simulink model "self_triggered_mpc_simulation"  (R2023a)
settings: Solver=VariableStepAuto  StartTime=0.0  StopTime=1  RelTol=1e-3
values from neighbouring files (symbols this model uses):
  param = param_setup()    [cost_cal.m]    (also in main.m; param.mat = ; self_triggered_mpc_heemels.m)
(part 1 of 2)
settings Model: Creator=김준수  LastModifiedBy=김준수
settings DebuggingCC: UnderSpecifiedDimensionMsg=error

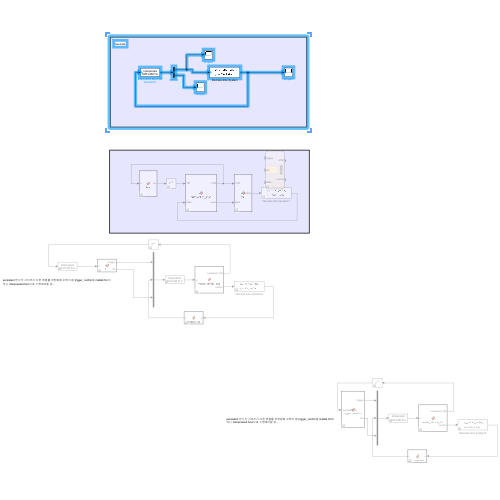
[thumbnail: Simulink's stored preview of the top-level diagram]
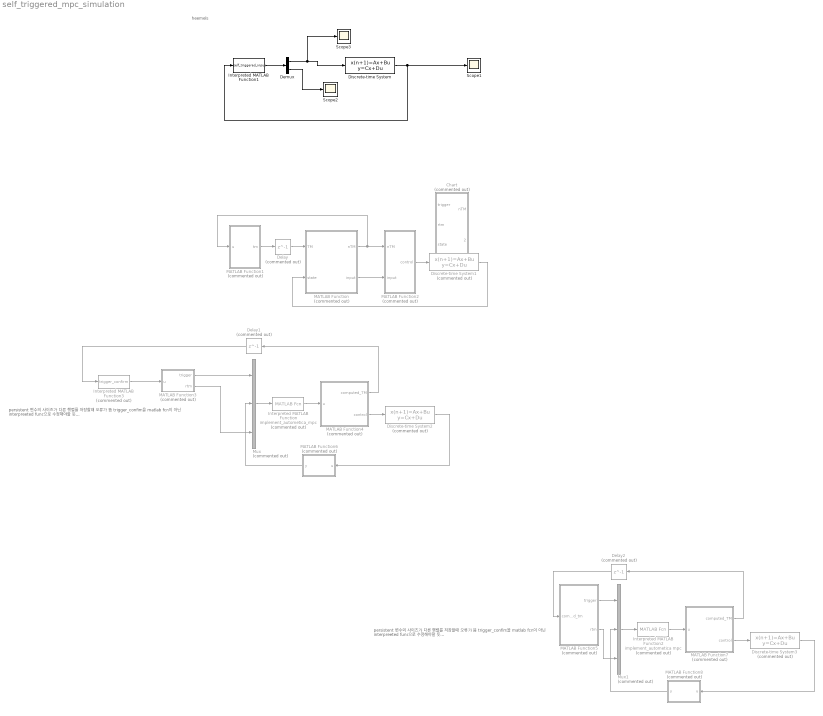
== system self_triggered_mpc_simulation ==
  note: persistent 변수의 사이즈가 다른 행렬를 저장할때 오류가 뜸 trigger_confim을 matlab fcn이 아닌 interpreeted func으로 수정해야할 듯...
  note: heemels
  note: persistent 변수의 사이즈가 다른 행렬를 저장할때 오류가 뜸 trigger_confim을 matlab fcn이 아닌 interpreeted func으로 수정해야할 듯...
  Chart : Stateflow chart  Commented=on  TreatAsAtomicUnit=on
  Delay : Delay  Commented=on  DelayLength=1
  Delay1 : Delay  Commented=on  DelayLength=1
  Delay2 : Delay  Commented=on  DelayLength=1
  Demux : Demux  Outputs=2
  Discrete-time System : DiscreteStateSpace  A=param.A  B=param.B  C=eye(param.nx)  D=zeros(param.nx,1)  InitialCondition=param.x0
  Discrete-time System1 : DiscreteStateSpace  Commented=on  A=param.A  B=param.B  C=eye(param.nx)  D=zeros(param.nx,1)  InitialCondition=param.x0
  Discrete-time System2 : DiscreteStateSpace  Commented=on  A=param.A  B=param.B  C=eye(param.nx)  D=zeros(param.nx,1)  InitialCondition=param.x0
  Discrete-time System3 : DiscreteStateSpace  Commented=on  A=param.A  B=param.B  C=eye(param.nx)  D=zeros(param.nx,1)  InitialCondition=param.x0
  Interpreted MATLAB Function : MATLABFcn  Commented=on  MATLABFcn=implement_autometica_mpc  Output1D=off
  Interpreted MATLAB Function1 : MATLABFcn  MATLABFcn=self_triggered_input  OutputDimensions=param.nu+1  Output1D=off
  Interpreted MATLAB Function2 : MATLABFcn  Commented=on  MATLABFcn=implement_autometica mpc
  Interpreted MATLAB Function3 : MATLABFcn  Commented=on  MATLABFcn=trigger_confirm  Output1D=off
  MATLAB Function : MATLAB Function  Commented=on  TreatAsAtomicUnit=on
  MATLAB Function1 : MATLAB Function  Commented=on  TreatAsAtomicUnit=on
  MATLAB Function2 : MATLAB Function  Commented=on  TreatAsAtomicUnit=on
  MATLAB Function3 : MATLAB Function  Commented=on  TreatAsAtomicUnit=on
  MATLAB Function4 : MATLAB Function  Commented=on  TreatAsAtomicUnit=on
  MATLAB Function5 : MATLAB Function  Commented=on  TreatAsAtomicUnit=on
  MATLAB Function6 : MATLAB Function  Commented=on  TreatAsAtomicUnit=on
  MATLAB Function7 : MATLAB Function  Commented=on  TreatAsAtomicUnit=on
  MATLAB Function8 : MATLAB Function  Commented=on  TreatAsAtomicUnit=on
  Mux : Mux  Commented=on  Inputs=3
  Mux1 : Mux  Commented=on  Inputs=3
  Scope1 : Scope
  Scope2 : Scope
  Scope3 : Scope
  wires:
  Discrete-time System/1 -> Scope1/1, Interpreted MATLAB Function1/1
  Interpreted MATLAB Function1/1 -> Demux/1
  Demux/1 -> Scope3/1, Discrete-time System/1
  Demux/2 -> Scope2/1
  MATLAB Function/1(nTM) -> MATLAB Function2/1(nTM), MATLAB Function1/1(u)
  Delay/1 -> MATLAB Function/1(TM)
  MATLAB Function1/1(tm) -> Delay/1
  MATLAB Function2/1(control) -> Discrete-time System1/1
  MATLAB Function/2(input) -> MATLAB Function2/2(input)
  Discrete-time System1/1 -> MATLAB Function/2(state)
  MATLAB Function3/1(trigger) -> Mux/1
  MATLAB Function3/2(rtm) -> Mux/3
  Delay1/1 -> Interpreted MATLAB Function3/1
  Mux/1 -> Interpreted MATLAB Function/1
  Interpreted MATLAB Function/1 -> MATLAB Function4/1(u)
  MATLAB Function4/1(computed_TM) -> Delay1/1
  MATLAB Function4/2(control) -> Discrete-time System2/1
  Discrete-time System2/1 -> MATLAB Function6/1(u)
  MATLAB Function6/1(y) -> Mux/2
  Interpreted MATLAB Function2/1 -> MATLAB Function7/1(u)
  Discrete-time System3/1 -> MATLAB Function8/1(u)
  MATLAB Function7/1(computed_TM) -> Delay2/1
  Delay2/1 -> MATLAB Function5/1(computed_tm)
  MATLAB Function5/1(trigger) -> Mux1/1
  MATLAB Function8/1(y) -> Mux1/2
  MATLAB Function5/2(rtm) -> Mux1/3
  Mux1/1 -> Interpreted MATLAB Function2/1
  MATLAB Function7/2(control) -> Discrete-time System3/1
  Interpreted MATLAB Function3/1 -> MATLAB Function3/1(u)

== matlab function self_triggered_mpc_simulation/MATLAB Function3 ==
  data: u input; trigger output; rtm output
function [trigger, rtm] = fcn(u)
    SizeOfu= size(u);
    trigger = u(1)
    rtm = u(2:SizeOfu(2))
end

== matlab function self_triggered_mpc_simulation/MATLAB Function4 ==
  data: computed_TM output; u input; control output
function [computed_TM, control] = vector_divide_fcn(u)
    control = u(1);
    computed_TM  = u(2:end);
end

== matlab function self_triggered_mpc_simulation/MATLAB Function5 ==
  data: computed_tm input; trigger output; rtm output
function [trigger, rtm] = trigger_confirm(computed_tm) 

%%이전 triggering step에서 계산된 computed_tm를 받아와서
%%현재의 required triggering time moment sequence(tm | computed_tm) 를 구하고 
%%self-triggered mpc 연산을 할 지 말지 결정하는 함수

    param = load("param.mat");
    param = param.param;
    
    SizeOfTM = size(computed_tm);
    persistent tm
    persistent last_trigger
    if isempty(tm)==1
        tm = [1 0 0 0 0 1];
    end
    if isempty(last_trigger) == 1
        last_trigger =0;
    end

    if last_trigger == 1
        tm = tm | computed_tm ;
    end
    
    if tm(1) == 0
        SizeOftm = size(tm);
        trigger = 0;
        temp = tm(2:SizeOftm(2));
        tm = temp;
        rtm = tm; %% nontrigger time 일때 trigger time moment는 사용되지 않는 쓰래기값이다. 
        last_trigger=0;
    elseif tm(1)==1
        SizeOftm = size(tm);
        trigger = 1;
        tm = tm(2:SizeOftm(2));
        if SizeOftm(2)-1>=param.M
            rtm = tm;
        else
            rtm = [tm zeros(1,param.M-1), 1];
        end
        last_trigger=1;
    end
end
% if tm(1) == 0
%     SizeOftm = size(tm);
%     trigger = 0;
%     tm = tm(2:SizeOftm(2));
%     rtm = tm; %% nontrigger time 일때 trigger time moment는 사용되지 않는 쓰래기값이다. 
% else
%

== matlab function self_triggered_mpc_simulation/MATLAB Function6 ==
  data: u input; y output
function y =trnaspose(u)

y = u';

== matlab function self_triggered_mpc_simulation/MATLAB Function7 ==
  data: computed_TM output; u input; control output
function [computed_TM, control] = vector_divide_fcn(u)
    SizeOfu=size(u);
    control = u(1:2);
    computed_TM  = u(3:SizeOfu(2));
end

== matlab function self_triggered_mpc_simulation/MATLAB Function8 ==
  data: u input; y output
function y =trnaspose(u)

y = u';

== matlab function self_triggered_mpc_simulation/MATLAB Function1 ==
  data: u input; tm output
function tm  = fcn(u)

y = u;

== matlab function self_triggered_mpc_simulation/MATLAB Function ==
  data: nTM output; input output; TM input; state input
function [nTM, input] = autometica_mpc(TM, state)

    coder.extrinsic("optimconstr", "optimproblem", "optimvar");
%==========================================================================
 %parameter setting
    param = load("param.mat");
    param = param.param;
    Nl = size(TM);
    param.N = Nl(2);
%==========================================================================
    %implement autometica vesion
    prob = optimproblem;
    x0 = optimvar('x0', param.nx);
    x = optimvar('x', param.nx, param.N);
    u0 = optimvar('u0', param.nu);
    u = optimvar('u',param.nu, (param.N)-1);
    size(u)
    cost_function =x0'*param.Q*x0+u0*param.R*u0;
    for i=1:param.N-1
        cost_function = cost_function + x(:,i)'*param.Q*x(:,i) + u(:,i)'*param.R*u(:,i); % terminal cost 설정해야 됨
    end
    prob.Objective = cost_function;
    
%==========================================================================
% model constraints

    model_constr = optimconstr(param.nx,(param.N)+1);
    model_constr(:,1) = x(:,1) == param.A*x0 + param.B*u0;
    for i=1:param.N-1
        model_constr(:,i+1) = x(:,i+1) == param.A*x(:,i) + param.B*u(:,i);
    end
    model_constr(:,(param.N)+1) = x0 == state;
    prob.Constraints.model_constr = model_constr;
    
%==========================================================================
%terminal set constraints
    constT = optimconstr(30,param.autometica_Tset+1);
       
    LL = param.tildeF - param.tildeG*param.tildeK;
    for i= 1:param.autometica_Tset
        constT(:,i) = LL*(param.A_BK^(i))*param.phi(:,1:2)*x(:,param.N)<=ones(30,1);
    end
    constT(1:param.NumOfConstr,param.autometica_Tset+1) = (param.F-param.G*param.K)*x(:,param.N)<=1;
    prob.Constraints.ConstT = constT;
%==========================================================================
% triggering constraints
    SizeOfTM = size(TM);
    tm = TM(2:SizeOfTM(2));
    SizeOftm = size(tm);
    tmcomp = find(tm);
    SizeOfTmcomp = size(tmcomp);
    % triggering_constr = optimconstr(param.N);
    % triggering_constr(1) = u0 == u(:,1);
    % for i = 1:param.N-2
    %     triggering_constr(i+1) = u(:,i)==u(:,i+1); %% i+1에서 triggering하면 u(:,i)~=u(:,i+1)
    % end
    % for i = 1:SizeOfTmcomp %% required triggering time moment setting
    %     if tmcomp(i)==1
    %         triggering_constr(tmcopm(i)) = u0 ~= u(:,1);
    %     else
    %         triggering_constr(tmcomp(i)) =  u(:,tmcomp(i)-1) ~= u(:,tmcomp(i));
    %     end
    % end
    nontm = find(~tm); 
    SizeOfnontm = size(nontm);
%==========================================================================
% required trigger time moment sequence에서 triggering time moment 추가하기
% 이부분에서 tmarr marker를 결과로 얻는데 tmarr는 triggering time moment sequence에서
% triggering time moment를 추가하여 얻을 수 있는 모든 sequence를 묶어 tmarr로 받는다

    tmarr = [];
    switch SizeOfnontm(2)
        case 9
            [tmarr, marker] = trigger_plus_9(tm);
        case 8
            [tmarr, marker] = trigger_plus_8(tm);
        case 7
            [tmarr, marker] = trigger_plus_7(tm);
        case 6
            [tmarr, marker] = trigger_plus_6(tm);
        case 5
            [tmarr, marker] = trigger_plus_5(tm);
        case 4
            [tmarr, marker] = trigger_plus_4(tm);
        case 3
            [tmarr, marker] = trigger_plus_3(tm);
        case 2
            [tmarr, marker] = trigger_plus_2(tm);
        case 1
            [tmarr, marker] = trigger_plus_1(tm);
        case 0
            [tmarr, marker] = trigger_plus_0(tm);
    end

%==========================================================================

    SizeOftmarr = size(tmarr);
    SizeOfmarker = size(marker);

    % triggering_constr = optimconstr(param.nu, SizeOftm(2));
    % triggering_constr(:,1) = u0 == u(:,1); %SizeOfTM == param.N
    % for i = 2:SizeOftm(2)
    %     triggering_constr(:,i) = u(:,i-1)==u(:,i); %% i+1에서 triggering하면 u(:,i)~=u(:,i+1)
    % end
    solArr = [];
    fvalArr = [];
    exitflagArr = [];
    for i = 1:SizeOfmarker(2)
        for j = marker(i):marker(i+1)-1 

            tm_setting = tmarr(j,:)
            triggering_constr = optimconstr(param.nu, SizeOftm(2));%tm이 정해짐

            for k = 1:SizeOftm(2) %% required triggering time moment setting
                k
                if  tm_setting(k) == 0
                    if k ==1
                        triggering_constr(:,k) = u0 == u(:,1) %%optimconstr에서 ~=가 지원되지 않음
                        show(triggering_constr(:,k))
                    else
                        size(triggering_constr(:,k))
                        size(u)
                        triggering_constr(:,k) =  u(:,k-1) == u(:,k)
                        show(triggering_constr(:,i))
                    end
                end
            end
            prob.Constraints.triggering_constr = triggering_constr
            [sol,fval,exitflag,output,lambda] = solve(prob)
            solArr = [solArr sol]
            fvalArr = [fvalArr fval]
            exitflagArr = [exitflagArr exitflag]
        end

        if ~isempty(exitflagArr==1)
            temp = min(fvalArr);
            [row, col] = find(fvalArr == temp);
            input=solArr(row, col).u0;
            nTM = tmarr(marker(i)+col-1,:);
            return;
        end
    end

end
    

    % prob.Constraints.triggering_constr = triggering_constr;
    % [sol,fval,exitflag,output,lambda] = solve(prob);
    % if exitflag == 1
    %     u = sol;
    %     t = tmcomp(1);
    %     nTM = tm(tmcomp(1)+1:SizeOftm)
% fevalArr = [];
%             
%             for c = 0:SizeOfnontmcomp %% 트리거 어디다 놓을지
%                 plustime = a
%                 while(1)
%                     tm(nontmcomp(c)) = 1;
                    
%                 for i = 1:SizeOfTmcomp %% required triggering time moment setting
%                     if tmcomp(i)==1
%                         triggering_constr(tmcopm(i)) = u0 ~= u(:,1);
%                     else
%                         triggering_constr(tmcomp(i)) =  u(:,tmcomp(i)-1) ~= u(:,tmcomp(i));
%                     end
%                 end
%                 [sol, fval, exitflag, output, lambda] = solve(prob);
               
%                 fevalArr = [feasible exitflag];
%                 fvalArr = [fvalArr, fval];
%                 solArr = [solArr, sol];
%             end
%             feasible = find(fevalArr,1);
%             if isempty(feasible) == 0
%                [row col]= min(fvalArr);
%                utemp = solarr(col);
%                u = utemp.u0;
%                ttemp =

== matlab function self_triggered_mpc_simulation/MATLAB Function2 ==
  data: nTM input; input input; control output
function control = fcn( nTM, input)
    persistent clk;
    persistent hold;
    if isempty(clk)==1
        hold = input;
        control = hold;
        clk = 1;
    else
        if (nTM)==0
            control = hold;
        else
            hold = input;
            control = hold;
            clk = 1;
        end
    end
end
